simulink model "mobile_robot_control"  (R2020a)
settings: Solver=ode4  StartTime=0.0  StopTime=15  FixedStep=0.1  RelTol=1e-3
undefined symbols (not defined in the file): kp1, kp2, L, theta_start, x_set, x_start, y_set, y_start
libraries: simulink x1
settings Model: Creator=krzysztof  LastModifiedBy=krzysztof

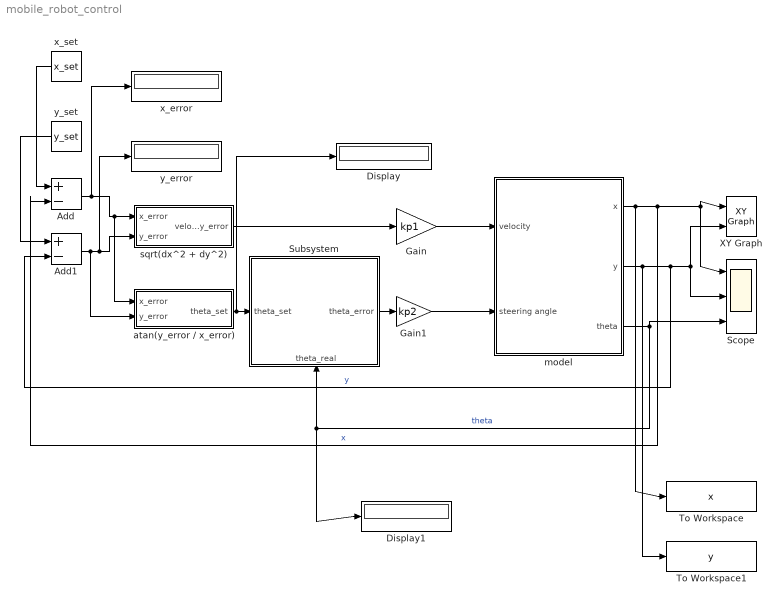
== system mobile_robot_control ==
  Add : Sum  Inputs=+-
  Add1 : Sum  Inputs=+-
  Display : Display
      settings: Format=short_e
  Display1 : Display
      settings: Format=short_e
  Gain : Gain  Gain=kp1
  Gain1 : Gain  Gain=kp2
  Scope : Scope  NumInputPorts=3
  Subsystem : Subsystem
      settings: PortSchema="{\"entries\":[{\"content\":{\"sides\":[{\"content\":{\"connectorIds\":[\"In1\"]},\"type\":\"ConnectorPlacement.EquallySpacedRectSide\",\"uuid\":\"fc3d2d42-6b75-4455-93d0-24c477eba1e2\"},{\"content\":{\"connectorIds\":[\"Out1\"],\"side\":\"RIGHT\"},\"type\":\"ConnectorPlacement.EquallySpacedRectSide\",\"uuid\":\"640ab7b6-8e5c-42d1-9d7a-31c2e9c3df8c\"},{\"content\":{\"connectorIds\":[],\"side\":\"TOP\"},\"type\":\"ConnectorPlacement.EquallySpacedRectSide\",\"uuid\":\"7c89bff5-0cce-42ff-a4c1-7cad39dc7ecc\"},{\"content\":{\"connectorIds\":[\"In2\"],\"side\":\"BOTTOM\"},\"type\":\"ConnectorPlacement.EquallySpacedRectSide\",\"uuid\":\"a37ec459-fa6b-4142-b403-d1bf8803b979\"}]},\"type\":\"ConnectorPlacement.EquallySpacedConnector\",\"uuid\":\"f605075b-9a69-4b03-9ecf-c2f7e2b5f79a\"}],\"packageUris\":[\"http://schema.mathworks.com/mf0/Connector/19700101\"],\"version\":\"1.0\"}"
  To Workspace : ToWorkspace  VariableName=x  SampleTime=-1
      settings: Save2DSignal=2-D array (concatenate along first dimension)
  To Workspace1 : ToWorkspace  VariableName=y  SampleTime=-1
      settings: Save2DSignal=2-D array (concatenate along first dimension)
  XY Graph : simulink/Sinks/XY Graph  xmin=0  xmax=10  ymin=0  ymax=10  st=-1
  atan(y_error / x_error) : Subsystem
  model : Subsystem
  sqrt(dx^2 + dy^2) : Subsystem
  x_error : Display
      settings: Format=short_e
  x_set : Constant  Value=x_set
  y_error : Display
      settings: Format=short_e
  y_set : Constant  Value=y_set
  wires:
  model/1(x) -> To Workspace/1, Add/2, XY Graph/1, Scope/1  "x"
  model/2(y) -> To Workspace1/1, Add1/2, XY Graph/2, Scope/2  "y"
  sqrt(dx^2 + dy^2)/1(velocity_error) -> Gain/1
  Gain/1 -> model/1(velocity)
  Gain1/1 -> model/2(steering angle)
  atan(y_error / x_error)/1(theta_set) -> Display/1, Subsystem/1(theta_set)
  Subsystem/1(theta_error) -> Gain1/1
  Add/1 -> x_error/1, atan(y_error / x_error)/1(x_error), sqrt(dx^2 + dy^2)/1(x_error)
  Add1/1 -> atan(y_error / x_error)/2(y_error), y_error/1, sqrt(dx^2 + dy^2)/2(y_error)
  x_set/1 -> Add/1
  y_set/1 -> Add1/1
  model/3(theta) -> Subsystem/2(theta_real), Display1/1, Scope/3  "theta"

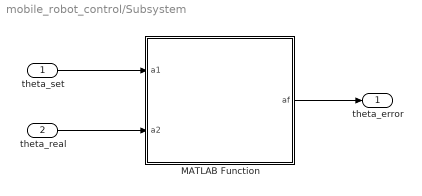
== system mobile_robot_control/Subsystem ==
  theta_set : Inport
  theta_real : Inport  Port=2
  MATLAB Function : MATLAB Function  TreatAsAtomicUnit=on
  theta_error : Outport
  wires:
  MATLAB Function/1(af) -> theta_error/1
  theta_set/1 -> MATLAB Function/1(a1)
  theta_real/1 -> MATLAB Function/2(a2)

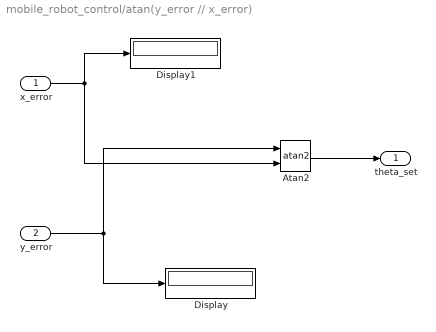
== system mobile_robot_control/atan(y_error // x_error) ==
  x_error : Inport
  y_error : Inport  Port=2
  Atan2 : Trigonometry  Operator=atan2
  Display : Display
      settings: Format=short_e
  Display1 : Display
      settings: Format=short_e
  theta_set : Outport
  wires:
  Atan2/1 -> theta_set/1
  x_error/1 -> Atan2/2, Display1/1
  y_error/1 -> Atan2/1, Display/1

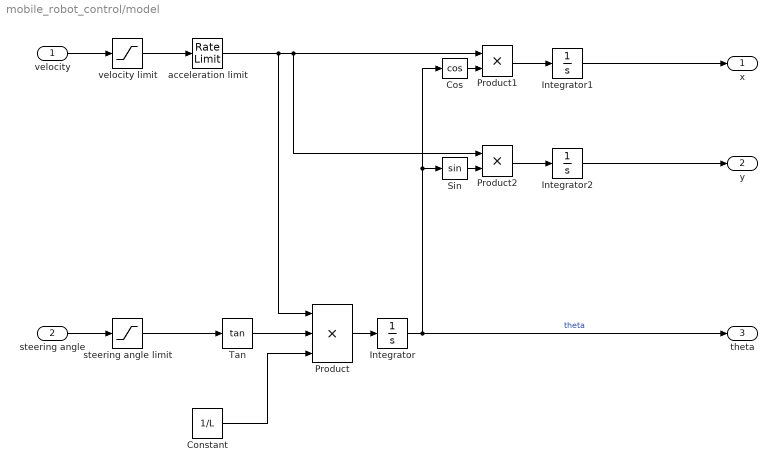
== system mobile_robot_control/model ==
  velocity : Inport
  steering angle : Inport  Port=2
  Constant : Constant  Value=1/L
  Cos : Trigonometry  Operator=cos  OutputSignalType=real
  Integrator : Integrator  InitialCondition=theta_start
  Integrator1 : Integrator  InitialCondition=x_start
  Integrator2 : Integrator  InitialCondition=y_start
  Product : Product  Inputs=3
  Product1 : Product
  Product2 : Product
  Sin : Trigonometry  OutputSignalType=real
  Tan : Trigonometry  Operator=tan
  acceleration limit : RateLimiter  SampleTimeMode=inherited
  steering angle limit : Saturate  UpperLimit=1  LowerLimit=-1  LinearizeAsGain=off
  velocity limit : Saturate  UpperLimit=2  LowerLimit=-2
  x : Outport
  y : Outport  Port=2
  theta : Outport  Port=3
  wires:
  Product1/1 -> Integrator1/1
  Integrator2/1 -> y/1
  Product2/1 -> Integrator2/1
  Integrator/1 -> theta/1, Cos/1, Sin/1  "theta"
  Integrator1/1 -> x/1
  Cos/1 -> Product1/2
  Tan/1 -> Product/2
  Constant/1 -> Product/3
  steering angle limit/1 -> Tan/1
  acceleration limit/1 -> Product/1, Product2/1, Product1/1
  Sin/1 -> Product2/2
  Product/1 -> Integrator/1
  steering angle/1 -> steering angle limit/1
  velocity limit/1 -> acceleration limit/1
  velocity/1 -> velocity limit/1

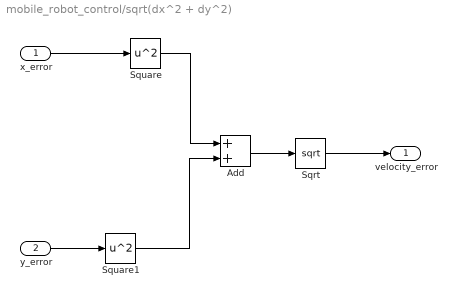
== system mobile_robot_control/sqrt(dx^2 + dy^2) ==
  x_error : Inport
  y_error : Inport  Port=2
  Add : Sum
  Sqrt : Sqrt  SaturateOnIntegerOverflow=on
  Square : Math  Operator=square  SaturateOnIntegerOverflow=on
  Square1 : Math  Operator=square  SaturateOnIntegerOverflow=on
  velocity_error : Outport
  wires:
  Sqrt/1 -> velocity_error/1
  x_error/1 -> Square/1
  y_error/1 -> Square1/1
  Square/1 -> Add/1
  Square1/1 -> Add/2
  Add/1 -> Sqrt/1

== matlab function mobile_robot_control/Subsystem/MATLAB Function ==
  data: a1 input; af output; a2 input
function af=angdif2(a1,a2)   % radians angles version
%
%   input : a1, a2
% output: af
a3=mod(a1-a2,2*pi);
af= 0;
q1=pi/2;
q2=pi;
q3=3*pi/2;
q4=2*pi;

if (0<a3)&&(a3<=q1)
    af=a3;
elseif (q1<a3)&&(a3<=q2) 
     af=a3;
elseif (q2<a3)&&(a3<=q3) 
    af=a3-q4;
elseif (q3<a3)&&(a3<=q4) 
    af= a3-q4;
elseif (-q1<=a3)&&(a3<0)    
    af=a3;
elseif (-q2<=a3)&&(a3<-q1) 
    af=a3;
elseif (-q3<=a3)&&(a3<-q2) 
    af =q4+a3;
elseif (-q4<=a3)&&(a3<-q3)
    af = q4+a3;
end

if af==pi af=-pi;
    
end

return
